simulink model "dfilter_3stage_fxpt_opt"  (Simulink 8.4)
settings: Solver=ode45  StartTime=0.0  StopTime=10.0  RelTol=1e-3
libraries: dspmlti4 x6, simulink_extras x1, simulink x1
settings Model: Creator=amatsumo  LastModifiedBy=kotsuka
settings DataIOCC: SaveOutput=off  SignalLogging=off  DSMLogging=off  SaveTime=off
settings OptimizationCC: BlockReduction=off  ConditionallyExecuteInputs=off  InlineParams=on
settings DebuggingCC: AlgebraicLoopMsg=error  SingleTaskRateTransMsg=error  FcnCallInpInsideContextMsg=EnableAllAsWarning
settings HardwareCC: ProdHWDeviceType=ASIC/FPGA->ASIC/FPGA  TargetLongLongMode=on  TargetIntDivRoundTo=Zero  TargetEndianess=LittleEndian  TargetHWDeviceType=MATLAB Host  ProdEqTarget=off

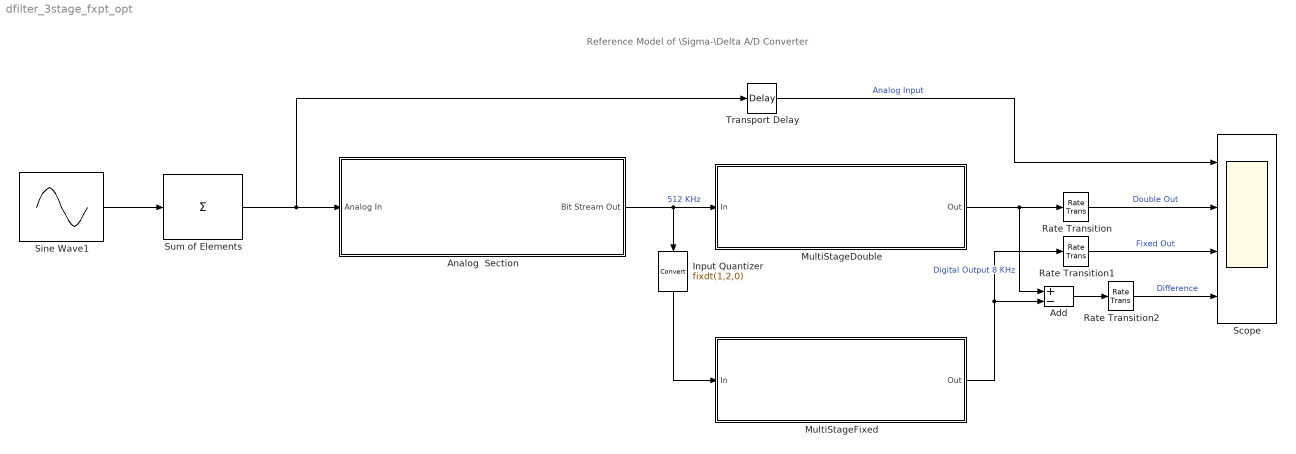
== system dfilter_3stage_fxpt_opt ==
  note: Reference Model of
      | \Sigma-\Delta A/D Converter
  Add : Sum  Inputs=+-
  Analog  Section : Subsystem
  Input Quantizer : DataTypeConversion  OutDataTypeStr=fixdt(1,2,0)  RndMeth=Round  SaturateOnIntegerOverflow=on
  MultiStageDouble : Subsystem  Tag=BlockMethodSubSystem
  MultiStageFixed : Subsystem  Tag=BlockMethodSubSystem
  Rate Transition : RateTransition
  Rate Transition1 : RateTransition
  Rate Transition2 : RateTransition
  Scope : Scope  NumInputPorts=4
      settings: TimeRange=0.0175  YMin=-1~-1~-0.75~-0.4  YMax=1~1~1~0.4
  Sine Wave1 : Sin  Amplitude=0.5  Frequency=2*pi*[1500 1750]  SampleTime=0
  Sum of Elements : Sum  Inputs=+
  Transport Delay : TransportDelay  DelayTime=(1/512e3*(31/2))+(8/512e3*(7/2))+(16/512e3*(121/2))
  wires:
  Analog  Section/1(Bit Stream Out) -> MultiStageDouble/1(In), Input Quantizer/1  "512 KHz"
  MultiStageDouble/1(Out) -> Add/1, Rate Transition/1  "Digital Output 8 KHz"
  Sum of Elements/1 -> Transport Delay/1, Analog  Section/1(Analog In)
  Sine Wave1/1 -> Sum of Elements/1
  Transport Delay/1 -> Scope/1  "Analog Input"
  MultiStageFixed/1(Out) -> Add/2, Rate Transition1/1
  Add/1 -> Rate Transition2/1
  Input Quantizer/1 -> MultiStageFixed/1(In)
  Rate Transition/1 -> Scope/2  "Double Out"
  Rate Transition1/1 -> Scope/3  "Fixed Out"
  Rate Transition2/1 -> Scope/4  "Difference"

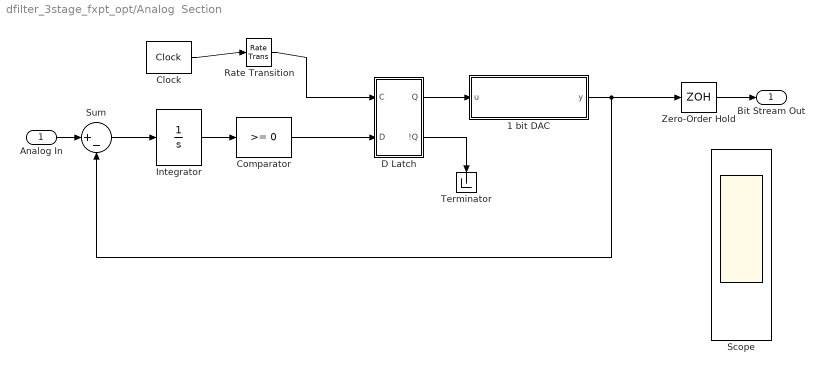
== system dfilter_3stage_fxpt_opt/Analog  Section ==
  Analog In : Inport
  1 bit DAC : MATLAB Function  TreatAsAtomicUnit=on
  Clock : simulink_extras/Flip Flops/Clock  period=1/512000
  Comparator : simulink/Logic and Bit Operations/Compare To Zero  relop=>=  OutDataTypeStr=boolean  ZeroCross=off
  D Latch : Subsystem  AncestorBlock=simulink_extras/Flip Flops/D Latch  mask(DLatch){}
      mask help: D Latch Flip-Flop Block
      mask Help:
      | The D latch flip-flop block has the following characteristic table:
      | <pre>
      |   Q(t)  D(t)     Q(tnext)
      |   ------------------------
      |    0      0       0
      |    0      1       1
      |    1      0       0
      |    1      1       1
      | </pre>
      | The D latch transfers "data" into a memory element (flip-flop).  The D latch
      | flip-flop is sometimes called a gated D-latch. The chip enable input signal, C,
      | is sometimes given the designation G (for gate) to indicate that this input
      | enables the gated latch allowing data entry into the flip-flop.
  Integrator : Integrator
  Rate Transition : RateTransition
  Scope : Scope  NumInputPorts=4
      settings: TimeRange=0.0175  YMin=-1~-1~-0.75~-0.4  YMax=1~1~1~0.4
  Sum : Sum  Inputs=|+-
  Terminator : Terminator
  Zero-Order Hold : ZeroOrderHold  SampleTime=1/512000
  Bit Stream Out : Outport
  wires:
  Sum/1 -> Integrator/1
  Integrator/1 -> Comparator/1
  D Latch/1(Q) -> 1 bit DAC/1(u)
  Comparator/1 -> D Latch/2(D)
  Clock/1 -> Rate Transition/1
  Analog In/1 -> Sum/1
  D Latch/2(!Q) -> Terminator/1
  1 bit DAC/1(y) -> Sum/2, Zero-Order Hold/1
  Zero-Order Hold/1 -> Bit Stream Out/1
  Rate Transition/1 -> D Latch/1(C)

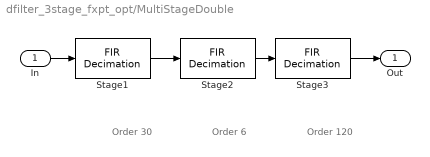
== system dfilter_3stage_fxpt_opt/MultiStageDouble ==
  note: Order 30
  note: Order 120
  note: Order 6
  In : Inport
  Stage1 : dspmlti4/FIR Decimation  Tag=BlockMethodSubSystem  h=[-0.00111887688497772 -0.00249700636744405 -0.00459514705449605 -0.00695605168661718 -0.00883309346046245 -0.00913347915153677 -0.00658179617561458 0 0.0113580022883622 0.0274930872781109 0.0474730357942702 0.0694361238436743 0.0908217187019734 0.108796639037714 0.120788011385266 0.125 0.120788011385266 0.108796639037714 0.0908217187019734 0.0694361238436743 0.0474730357942702 0.0274930872781109 0.0113580022883622 0 -0.00658179617561458 -0.00913347915153677 -0.00883309346046245 -0.00695605168661718 -0.00459514705449605 -0.00249700636744405 -0.00111887688497772]  D=8  filtStruct=Direct form  framing=Allow multirate processing  inputOffset=0  outputBufInitCond=0  firstCoeffDataTypeStr=Inherit: Same word length as input  firstCoeffLastDataTypeStr=Inherit: Same word length as input  firstCoeffMin=[]  firstCoeffMax=[]  outputDataTypeStr=Inherit: Same as accumulator  outputLastDataTypeStr=Inherit: Same as accumulator  outputMin=[]  outputMax=[]  roundingMode=Floor  overflowMode=off  FilterSource=Specify via dialog  FilterObject=Hm_firdecim
      settings: allowOverrides=off
  Stage2 : dspmlti4/FIR Decimation  Tag=BlockMethodSubSystem  h=[-0.0362429732032996 0 0.285766556113462 0.5 0.285766556113462 0 -0.0362429732032996]  D=2  filtStruct=Direct form  framing=Allow multirate processing  inputOffset=0  outputBufInitCond=0  firstCoeffDataTypeStr=Inherit: Same word length as input  firstCoeffLastDataTypeStr=Inherit: Same word length as input  firstCoeffMin=[]  firstCoeffMax=[]  outputDataTypeStr=Inherit: Same as accumulator  outputLastDataTypeStr=Inherit: Same as accumulator  outputMin=[]  outputMax=[]  roundingMode=Floor  overflowMode=off  FilterSource=Specify via dialog  FilterObject=Hm_firdecim
      settings: allowOverrides=off
  Stage3 : dspmlti4/FIR Decimation  Tag=BlockMethodSubSystem  h=[0 8.47606608023409e-005 0.000153854327095139 0.000136317924712582 0 -0.00020305751735692 -0.00034351785801204 -0.000287512764448896 0 0.000392439332338858 0.000641352526162708 0.000520829654785754 0 -0.000675934489470505 -0.00108130615140325 -0.000861294784663789 0 0.00108078812901365 0.00170363859454544 0.00133869559937353 0 -0.00163979704643895 -0.00255719195777936 -0.00198950613899863 0 0.00239406143369657 0.00370403184027956 0.00286079736392912 0 -0.00339853108587054 -0.00522879369788111 -0.00401812063684183 0 0.00473328239621661 0.00725782810372907 0.00556181181617326 0 -0.00652745120402357 -0.0100005039196451 -0.00766283375033631 0 0.00901429412175636 0.0138468308039176 0.0106500795049504 0 -0.0126751309317764 -0.0196334619787484 -0.0152595059298061 0 0.0186977987055184 0.0295485536348429 0.0235477697350464 0 -0.0310065956743577 -0.0516550323392064 -0.0441900663694138 0 0.0745284672846225 0.158684803330616 0.224912706095971 0.25 0.224912706095971 0.158684803330616 0.0745284672846225 0 -0.0441900663694138 -0.0516550323392064 -0.0310065956743577 0 0.0235477697350464 0.0295485536348429 0.0186977987055184 0 -0.0152595059298061 -0.0196334619787484 -0.0126751309317764 0 0.0106500795049504 0.0138468308039176 0.00901429412175636 0 -0.00766283375033631 -0.0100005039196451 -0.00652745120402357 0 0.00556181181617326 0.00725782810372907 0.00473328239621661 0 -0.00401812063684183 -0.00522879369788111 -0.00339853108587054 0 0.00286079736392912 0.00370403184027956 0.00239406143369657 0 -0.00198950613899863 -0.00255719195777936 -0.00163979704643895 0 0.00133869559937353 0.00170363859454544 0.00108078812901365 0 -0.000861294784663789 -0.00108130615140325 -0.000675934489470505 0 0.000520829654785754 0.000641352526162708 0.000392439332338858 0 -0.000287512764448896 -0.00034351785801204 -0.00020305751735692 0 0.000136317924712582 0.000153854327095139 8.47606608023409e-005 0]  D=4  filtStruct=Direct form  framing=Allow multirate processing  inputOffset=0  outputBufInitCond=0  firstCoeffDataTypeStr=Inherit: Same word length as input  firstCoeffLastDataTypeStr=Inherit: Same word length as input  firstCoeffMin=[]  firstCoeffMax=[]  outputDataTypeStr=Inherit: Same as accumulator  outputLastDataTypeStr=Inherit: Same as accumulator  outputMin=[]  outputMax=[]  roundingMode=Floor  overflowMode=off  FilterSource=Specify via dialog  FilterObject=Hm_firdecim
      settings: allowOverrides=off
  Out : Outport
  wires:
  In/1 -> Stage1/1
  Stage1/1 -> Stage2/1
  Stage2/1 -> Stage3/1
  Stage3/1 -> Out/1

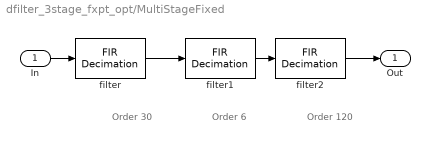
== system dfilter_3stage_fxpt_opt/MultiStageFixed ==
  note: Order 30
  note: Order 120
  note: Order 6
  In : Inport
  filter : dspmlti4/FIR Decimation  h=[-0.00112152099609375 -0.00249481201171875 -0.0045928955078125 -0.0069580078125 -0.0088348388671875 -0.00913238525390625 -0.00658416748046875 0 0.0113601684570313 0.027496337890625 0.0474700927734375 0.0694351196289063 0.0908203125 0.108795166015625 0.12078857421875 0.125 0.12078857421875 0.108795166015625 0.0908203125 0.0694351196289063 0.0474700927734375 0.027496337890625 0.0113601684570313 0 -0.00658416748046875 -0.00913238525390625 -0.0088348388671875 -0.0069580078125 -0.0045928955078125 -0.00249481201171875 -0.00112152099609375]  D=8  filtStruct=Direct form  framing=Allow multirate processing  inputOffset=0  outputBufInitCond=0  firstCoeffMode=Binary point scaling  firstCoeffWordLength=16  firstCoeffFracLength=17  firstCoeffDataTypeStr=fixdt(1,16,17)  firstCoeffLastDataTypeStr=fixdt(1,16,17)  firstCoeffMin=[]  firstCoeffMax=[]  outputMode=Binary point scaling  outputWordLength=17  outputFracLength=15  outputDataTypeStr=fixdt(1,17,15)  outputLastDataTypeStr=fixdt(1,17,15)  outputMin=[]  outputMax=[]  accumMode=Binary point scaling  accumWordLength=31  accumFracLength=29  accumDataTypeStr=fixdt(1,31,29)  accumLastDataTypeStr=fixdt(1,31,29)  prodOutputMode=Binary point scaling  prodOutputWordLength=28  prodOutputFracLength=29  prodOutputDataTypeStr=fixdt(1,28,29)  prodOutputLastDataTypeStr=fixdt(1,28,29)  roundingMode=Convergent  overflowMode=off  FilterSource=Specify via dialog  FilterObject=Hm_firdecim
      settings: allowOverrides=off
  filter1 : dspmlti4/FIR Decimation  h=[-0.0362548828125 0 0.2857666015625 0.5 0.2857666015625 0 -0.0362548828125]  D=2  filtStruct=Direct form  framing=Allow multirate processing  inputOffset=0  outputBufInitCond=0  firstCoeffMode=Binary point scaling  firstCoeffWordLength=16  firstCoeffFracLength=15  firstCoeffDataTypeStr=fixdt(1,16,15)  firstCoeffLastDataTypeStr=fixdt(1,16,15)  firstCoeffMin=[]  firstCoeffMax=[]  outputMode=Binary point scaling  outputWordLength=17  outputFracLength=15  outputDataTypeStr=fixdt(1,17,15)  outputLastDataTypeStr=fixdt(1,17,15)  outputMin=[]  outputMax=[]  accumMode=Binary point scaling  accumWordLength=31  accumFracLength=29  accumDataTypeStr=fixdt(1,31,29)  accumLastDataTypeStr=fixdt(1,31,29)  prodOutputMode=Binary point scaling  prodOutputWordLength=30  prodOutputFracLength=29  prodOutputDataTypeStr=fixdt(1,30,29)  prodOutputLastDataTypeStr=fixdt(1,30,29)  roundingMode=Convergent  overflowMode=off  FilterSource=Specify via dialog  FilterObject=Hm_firdecim
      settings: allowOverrides=off
  filter2 : dspmlti4/FIR Decimation  h=[0 9.1552734375e-005 0.000152587890625 0.0001373291015625 0 -0.0001983642578125 -0.0003509521484375 -0.0002899169921875 0 0.000396728515625 0.000640869140625 0.000518798828125 0 -0.00067138671875 -0.0010833740234375 -0.0008544921875 0 0.0010833740234375 0.001708984375 0.0013427734375 0 -0.0016326904296875 -0.0025634765625 -0.001983642578125 0 0.0023956298828125 0.0037078857421875 0.0028533935546875 0 -0.0034027099609375 -0.0052337646484375 -0.0040130615234375 0 0.004730224609375 0.00726318359375 0.00555419921875 0 -0.00653076171875 -0.0099945068359375 -0.007659912109375 0 0.0090179443359375 0.0138397216796875 0.010650634765625 0 -0.0126800537109375 -0.0196380615234375 -0.0152587890625 0 0.0186920166015625 0.029541015625 0.0235443115234375 0 -0.031005859375 -0.0516510009765625 -0.044189453125 0 0.07452392578125 0.15869140625 0.22491455078125 0.25 0.22491455078125 0.15869140625 0.07452392578125 0 -0.044189453125 -0.0516510009765625 -0.031005859375 0 0.0235443115234375 0.029541015625 0.0186920166015625 0 -0.0152587890625 -0.0196380615234375 -0.0126800537109375 0 0.010650634765625 0.0138397216796875 0.0090179443359375 0 -0.007659912109375 -0.0099945068359375 -0.00653076171875 0 0.00555419921875 0.00726318359375 0.004730224609375 0 -0.0040130615234375 -0.0052337646484375 -0.0034027099609375 0 0.0028533935546875 0.0037078857421875 0.0023956298828125 0 -0.001983642578125 -0.0025634765625 -0.0016326904296875 0 0.0013427734375 0.001708984375 0.0010833740234375 0 -0.0008544921875 -0.0010833740234375 -0.00067138671875 0 0.000518798828125 0.000640869140625 0.000396728515625 0 -0.0002899169921875 -0.0003509521484375 -0.0001983642578125 0 0.0001373291015625 0.000152587890625 9.1552734375e-005 0]  D=4  filtStruct=Direct form  framing=Allow multirate processing  inputOffset=0  outputBufInitCond=0  firstCoeffMode=Binary point scaling  firstCoeffWordLength=16  firstCoeffFracLength=16  firstCoeffDataTypeStr=fixdt(1,16,16)  firstCoeffLastDataTypeStr=fixdt(1,16,16)  firstCoeffMin=[]  firstCoeffMax=[]  outputMode=Binary point scaling  outputWordLength=16  outputFracLength=14  outputDataTypeStr=fixdt(1,16,14)  outputLastDataTypeStr=fixdt(1,16,14)  outputMin=[]  outputMax=[]  accumMode=Binary point scaling  accumWordLength=30  accumFracLength=28  accumDataTypeStr=fixdt(1,30,28)  accumLastDataTypeStr=fixdt(1,30,28)  prodOutputMode=Binary point scaling  prodOutputWordLength=29  prodOutputFracLength=29  prodOutputDataTypeStr=fixdt(1,29,29)  prodOutputLastDataTypeStr=fixdt(1,29,29)  roundingMode=Convergent  overflowMode=off  FilterSource=Specify via dialog  FilterObject=Hm_firdecim
      settings: allowOverrides=off
  Out : Outport
  wires:
  filter2/1 -> Out/1
  filter1/1 -> filter2/1
  filter/1 -> filter1/1
  In/1 -> filter/1

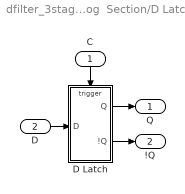
== system dfilter_3stage_fxpt_opt/Analog  Section/D Latch ==
  C : Inport
  D : Inport  Port=2
  D Latch : Subsystem  TreatAsAtomicUnit=on
  Q : Outport  InitialOutput=0
  !Q : Outport  Port=2  InitialOutput=1
  wires:
  C/1 -> D Latch/Trigger
  D Latch/1(Q) -> Q/1
  D/1 -> D Latch/1(D)
  D Latch/2(!Q) -> !Q/1

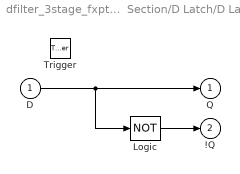
== system dfilter_3stage_fxpt_opt/Analog  Section/D Latch/D Latch ==
  D : Inport
  Trigger : TriggerPort  StatesWhenEnabling=reset
  Logic : Logic  Operator=NOT  Inputs=1
  Q : Outport  InitialOutput=0
  !Q : Outport  Port=2  InitialOutput=1
  wires:
  Logic/1 -> !Q/1
  D/1 -> Q/1, Logic/1

== matlab function Analog Section/1 bit DAC ==
  data: u input double; y output double
function y = DAC_1_bit(u)
% This block supports an embeddable subset of the MATLAB language.
% See the help menu for details.

% This code converts boolean input to a bipolar output (double precision). 

y=-1+2*u;
